simulink model "Aircraft6DOFTrim"  (R2022a)
settings: Solver=VariableStepAuto  StartTime=0.0  StopTime=300  FixedStep=0.5  RelTol=1e-3
undefined symbols (not defined in the file): a0, a1, a2, a3, ac, alpha0, alpha_stall, c, cbar, cg, CLa, delta_aileronMax, delta_aileronMin, delta_elevatorMax, delta_elevatorMin, delta_rudderMax, delta_rudderMin, delta_thrustMax, delta_thrustMin, depsilon, Earth, engArm1, engArm2, falling_slew_rate, h_ref, Lat0, Lon0, LT, mass, rising_slew_rate, S, ST, WGS84, x
libraries: aerolibasang x3, aerolibfltsims x2, aerolibatmos2 x1, aerolibtransform2 x1
settings Model: Creator=wangL  LastModifiedBy=wangL
settings DataIOCC: ExternalInput=U_trim.getElement(1),U_trim.getElement(2),U_trim.getElement(3),U_trim.getElement(4),U_trim.getElement(5)

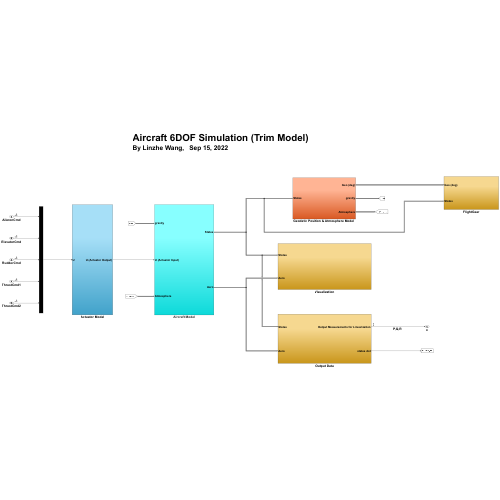
[thumbnail: Simulink's stored preview of the top-level diagram]
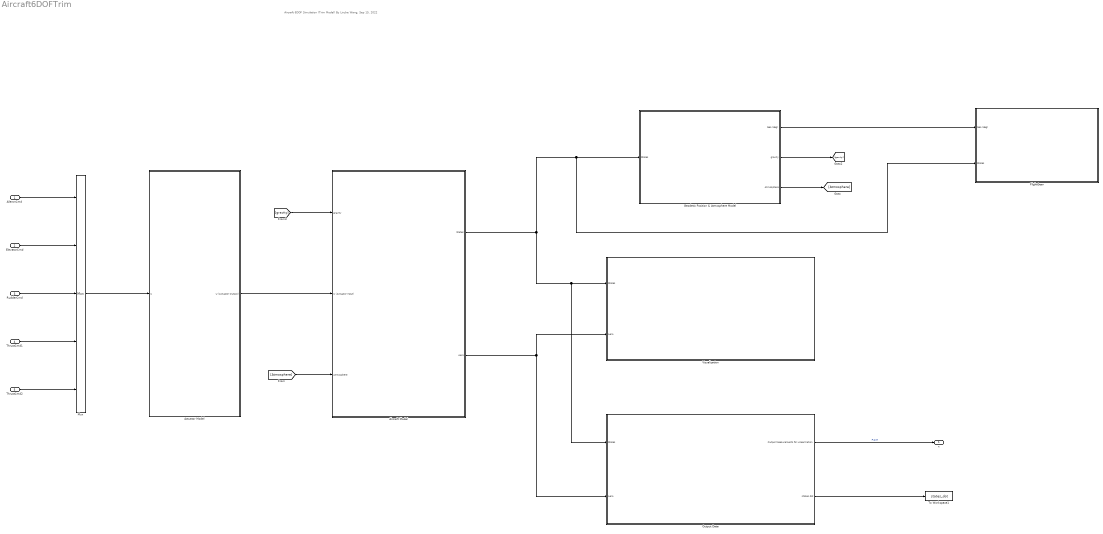
== system Aircraft6DOFTrim ==
  note: Aircraft 6DOF Simulation (Trim Model)
      | By Linzhe Wang, Sep 15, 2022
  AileronCmd : Inport
  ElevatorCmd : Inport  Port=2
  RudderCmd : Inport  Port=3
  ThrustCmd1 : Inport  Port=4
  ThrustCmd2 : Inport  Port=5
  Actuator Model : Subsystem
  Aircraft Model : Subsystem
  FlightGear : Subsystem
  "Geodetic Position & Atmosphere Model " : Subsystem
  Mux : Mux  Inputs=5
  Output Data : Subsystem
  To Workspace1 : ToWorkspace  VariableName=states_dot  SaveFormat=Structure With Time  SampleTime=-1
      settings: MaxDataPoints=1
  Visualization : Subsystem
  x : Outport
  wires:
  "Geodetic Position & Atmosphere Model "/1(Geo (deg)) -> FlightGear/1(Geo (deg))
  "Geodetic Position & Atmosphere Model "/2(gravity) -> [gravity]
  [gravity] -> Aircraft Model/1(gravity)
  Actuator Model/1(U (Actuator Output)) -> Aircraft Model/2(U (Actuator Input))
  "Geodetic Position & Atmosphere Model "/3(Atmosphere) -> [Atmosphere]
  [Atmosphere] -> Aircraft Model/3(Atmosphere)
  ElevatorCmd/1 -> Mux/2
  ThrustCmd2/1 -> Mux/5
  ThrustCmd1/1 -> Mux/4
  Mux/1 -> Actuator Model/1(U)
  RudderCmd/1 -> Mux/3
  AileronCmd/1 -> Mux/1
  Output Data/1(Output Measurements for Linearization) -> x/1  "P,Q,R"
  Output Data/2(states dot) -> To Workspace1/1
  Aircraft Model/1(States) -> Output Data/1(States), Visualization/1(States), "Geodetic Position & Atmosphere Model "/1(States), FlightGear/2(States)
  Aircraft Model/2(Aero) -> Output Data/2(Aero), Visualization/2(Aero)

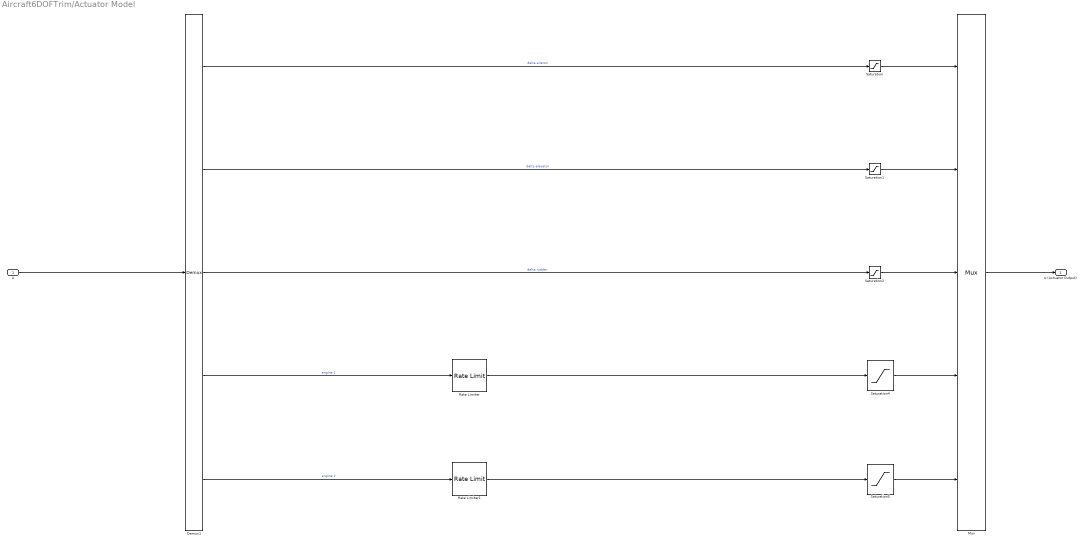
== system Aircraft6DOFTrim/Actuator Model ==
  U : Inport
  Demux1 : Demux  Outputs=5
  Mux : Mux  Inputs=5
  Rate Limiter : RateLimiter  RisingSlewLimit=rising_slew_rate  FallingSlewLimit=falling_slew_rate  SampleTimeMode=inherited
  Rate Limiter1 : RateLimiter  RisingSlewLimit=rising_slew_rate  FallingSlewLimit=falling_slew_rate  SampleTimeMode=inherited
  Saturation : Saturate  UpperLimit=delta_aileronMax  LowerLimit=delta_aileronMin
  Saturation1 : Saturate  UpperLimit=delta_elevatorMax  LowerLimit=delta_elevatorMin
  Saturation2 : Saturate  UpperLimit=delta_rudderMax  LowerLimit=delta_rudderMin
  Saturation4 : Saturate  UpperLimit=delta_thrustMax  LowerLimit=delta_thrustMin
  Saturation5 : Saturate  UpperLimit=delta_thrustMax  LowerLimit=delta_thrustMin
  U (Actuator Output) : Outport
  wires:
  Demux1/3 -> Saturation2/1  "delta rudder"
  Demux1/5 -> Rate Limiter1/1  "engine 2"
  Saturation4/1 -> Mux/4
  Saturation5/1 -> Mux/5
  Mux/1 -> U (Actuator Output)/1
  Demux1/2 -> Saturation1/1  "delta elevator"
  Demux1/1 -> Saturation/1  "delta aileron"
  Saturation/1 -> Mux/1
  Saturation1/1 -> Mux/2
  Saturation2/1 -> Mux/3
  Demux1/4 -> Rate Limiter/1  "engine 1"
  Rate Limiter1/1 -> Saturation5/1
  Rate Limiter/1 -> Saturation4/1
  U/1 -> Demux1/1

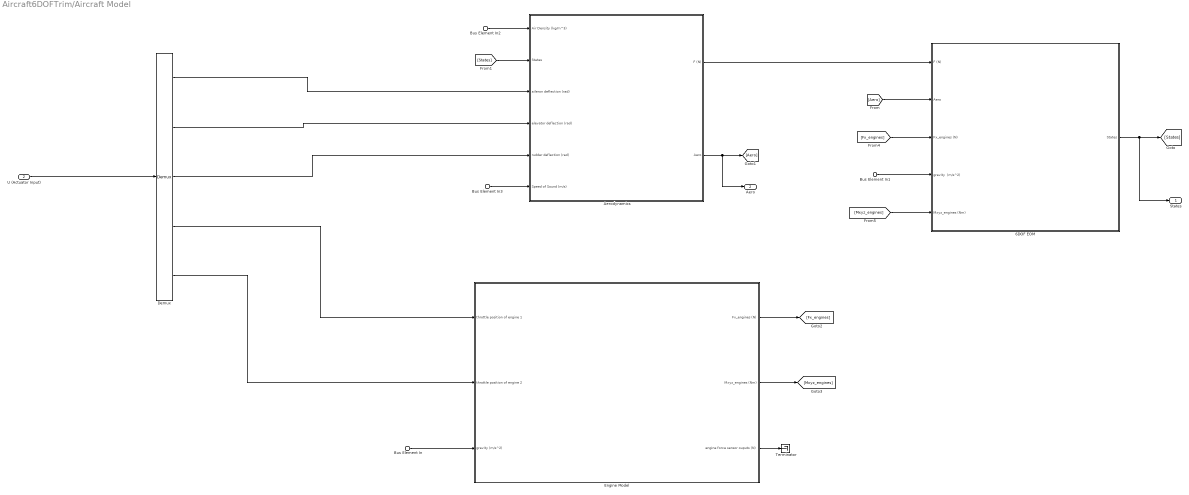
== system Aircraft6DOFTrim/Aircraft Model ==
  Bus Element In : Inport  PortName=gravity  Element=m/s^2
  Bus Element In1 : Inport  PortName=gravity  Element=m/s^2
  U (Actuator Input) : Inport  Port=2
  Bus Element In2 : Inport  Port=3  PortName=Atmosphere  Element=rho
  Bus Element In3 : Inport  Port=3  PortName=Atmosphere  Element=speedOfSound
  6DOF EOM : Subsystem
  Aerodynamics : Subsystem
  Demux : Demux  Outputs=5
  "Engine Model " : Subsystem
  Terminator : Terminator
  States : Outport
  Aero : Outport  Port=2
  wires:
  [Fx_engines] -> 6DOF EOM/3(Fx_engines (N))
  [Mxyz_engines] -> 6DOF EOM/5("Mxyz_engines (Nm) ")
  Aerodynamics/1(F (N)) -> 6DOF EOM/1(F (N))
  6DOF EOM/1(States) -> States/1, [States]
  "Engine Model "/1(Fx_engines (N)) -> [Fx_engines]
  "Engine Model "/2("Mxyz_engines (Nm) ") -> [Mxyz_engines]
  Aerodynamics/2(Aero) -> Aero/1, [Aero]
  [States] -> Aerodynamics/2(States)
  [Aero] -> 6DOF EOM/2(Aero)
  U (Actuator Input)/1 -> Demux/1
  Bus Element In/1 -> "Engine Model "/3(gravity (m/s^2))
  Bus Element In1/1 -> 6DOF EOM/4(gravity  (m/s^2))
  "Engine Model "/3(engine force sensor ouputs (N)) -> Terminator/1
  Demux/1 -> Aerodynamics/3(aileron deflection (rad))
  Demux/2 -> Aerodynamics/4(" elevator deflection (rad)")
  Demux/3 -> Aerodynamics/5(rudder deflection (rad))
  Demux/4 -> "Engine Model "/1(throttle position of engine 1)
  Demux/5 -> "Engine Model "/2(throttle position of engine 2)
  Bus Element In2/1 -> Aerodynamics/1(Air Density (kg/m^3))
  Bus Element In3/1 -> Aerodynamics/6(Speed of Sound (m/s))

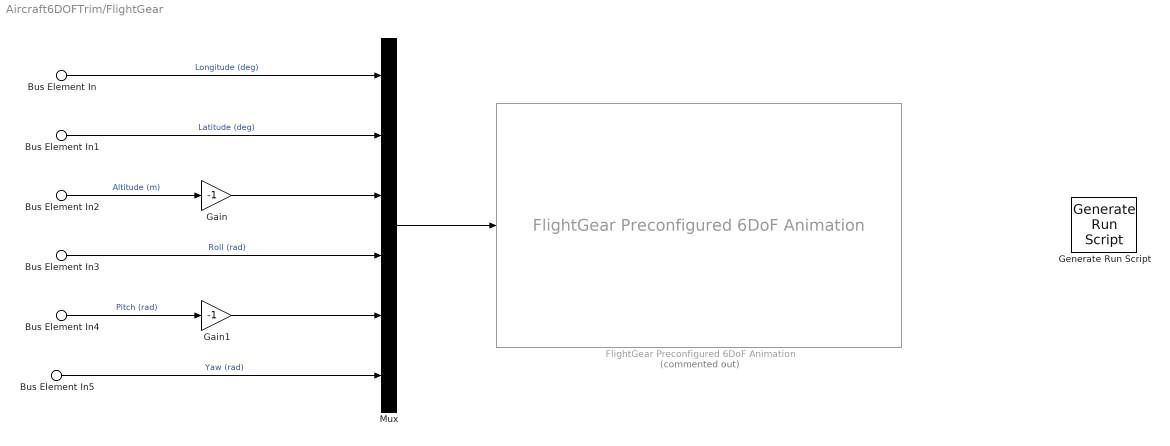
== system Aircraft6DOFTrim/FlightGear ==
  Bus Element In : Inport  PortName=Geo (deg)  Element=Lon
  Bus Element In1 : Inport  PortName=Geo (deg)  Element=Lat
  Bus Element In2 : Inport  Port=2  PortName=States  Element=h
  Bus Element In3 : Inport  Port=2  PortName=States  Element=phi
  Bus Element In4 : Inport  Port=2  PortName=States  Element=theta
  Bus Element In5 : Inport  Port=2  PortName=States  Element=psi
  FlightGear Preconfigured 6DoF Animation : aerolibfltsims/FlightGear Preconfigured 6DoF Animation  Commented=on  xFlightGearVersion=v2019.1  DestinationIpAddress=127.0.0.1  DestinationPort=5502  SampleTime=1/30  packetVersion=24
  Gain : Gain  Gain=-1
  Gain1 : Gain  Gain=-1
  Generate Run Script : aerolibfltsims/Generate Run Script  Architecture=Win64  dataFlow=Send  GeometryModelName=738  AirportId=KSFO  RunwayId=10L  InitialAltitude=0  InitialHeading=0  OffsetDistance=0  OffsetAzimuth=0  InstallScenery=off  DisableShaders=on  OriginAddress=127.0.0.1  DestinationPort=5502  OriginPort=5505  LocalAddress=127.0.0.1  OutputFileName=runfg.bat  FlightGearBaseDirectory=C:\Program Files\FlightGear 2020.3
  Mux : Mux  Inputs=6
  wires:
  Mux/1 -> FlightGear Preconfigured 6DoF Animation/1
  Bus Element In/1 -> Mux/1  "Longitude (deg)"
  Bus Element In1/1 -> Mux/2  "Latitude (deg)"
  Bus Element In2/1 -> Gain/1  "Altitude (m)"
  Bus Element In3/1 -> Mux/4  "Roll (rad)"
  Bus Element In4/1 -> Gain1/1  "Pitch (rad)"
  Bus Element In5/1 -> Mux/6  "Yaw (rad)"
  Gain/1 -> Mux/3
  Gain1/1 -> Mux/5

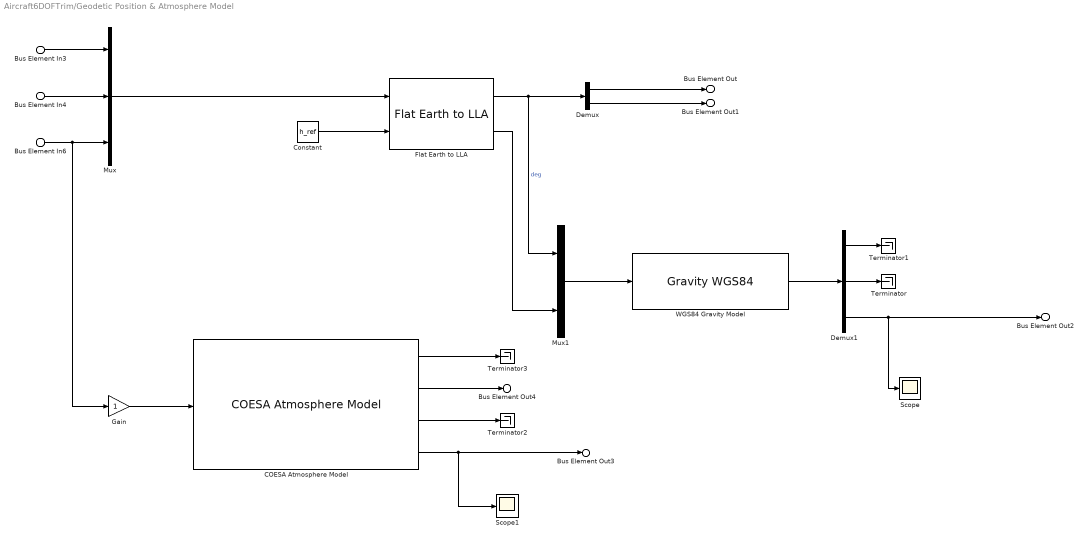
== system Aircraft6DOFTrim/Geodetic Position & Atmosphere Model  ==
  Bus Element In3 : Inport  PortName=States  Element=PN
  Bus Element In4 : Inport  PortName=States  Element=PE
  Bus Element In6 : Inport  PortName=States  Element=h
  COESA Atmosphere Model : aerolibatmos2/COESA Atmosphere Model  units=Metric (MKS)  spec=1976 COESA-extended U.S. Standard Atmosphere  model=Profile  profile_var=High temperature  profile_percent=1%  profile_alt=5 km (16404 ft)  envelope_var=High temperature  envelope_percent=1%  action=None
  Constant : Constant  Value=h_ref
  Demux : Demux  Outputs=2
  Demux1 : Demux  Outputs=3
  Flat Earth to LLA : aerolibtransform2/Flat Earth to LLA  units=Metric (MKS)  ptype=Earth (WGS84)  F=1/298.257223563  R=6378137  refPosPort=off  LL0=[Lat0 Lon0]  psi=0
  Gain : Gain
  Mux : Mux  Inputs=3
  Mux1 : Mux  Inputs=2
  Scope : Scope
  Scope1 : Scope
  Terminator{,1..3} (4 alike) : Terminator
  "WGS84 Gravity Model  " : GravityWGS84  action=None
  Bus Element Out : Outport  PortName=Geo (deg)  Element=Lat
  Bus Element Out1 : Outport  PortName=Geo (deg)  Element=Lon
  Bus Element Out2 : Outport  Port=2  PortName=gravity  Element=m/s^2
  Bus Element Out3 : Outport  Port=3  PortName=Atmosphere  Element=rho
  Bus Element Out4 : Outport  Port=3  PortName=Atmosphere  Element=speedOfSound
  wires:
  Constant/1 -> Flat Earth to LLA/2
  Bus Element In3/1 -> Mux/1
  Bus Element In4/1 -> Mux/2
  Bus Element In6/1 -> Mux/3, Gain/1
  Flat Earth to LLA/1 -> Demux/1, Mux1/1  "deg"
  Demux/1 -> Bus Element Out/1
  Demux/2 -> Bus Element Out1/1
  Mux/1 -> Flat Earth to LLA/1
  Mux1/1 -> "WGS84 Gravity Model  "/1
  Flat Earth to LLA/2 -> Mux1/2
  "WGS84 Gravity Model  "/1 -> Demux1/1
  Demux1/2 -> Terminator/1
  Demux1/1 -> Terminator1/1
  Demux1/3 -> Bus Element Out2/1, Scope/1
  COESA Atmosphere Model/2 -> Bus Element Out4/1
  COESA Atmosphere Model/3 -> Terminator2/1
  COESA Atmosphere Model/1 -> Terminator3/1
  Gain/1 -> COESA Atmosphere Model/1
  COESA Atmosphere Model/4 -> Bus Element Out3/1, Scope1/1

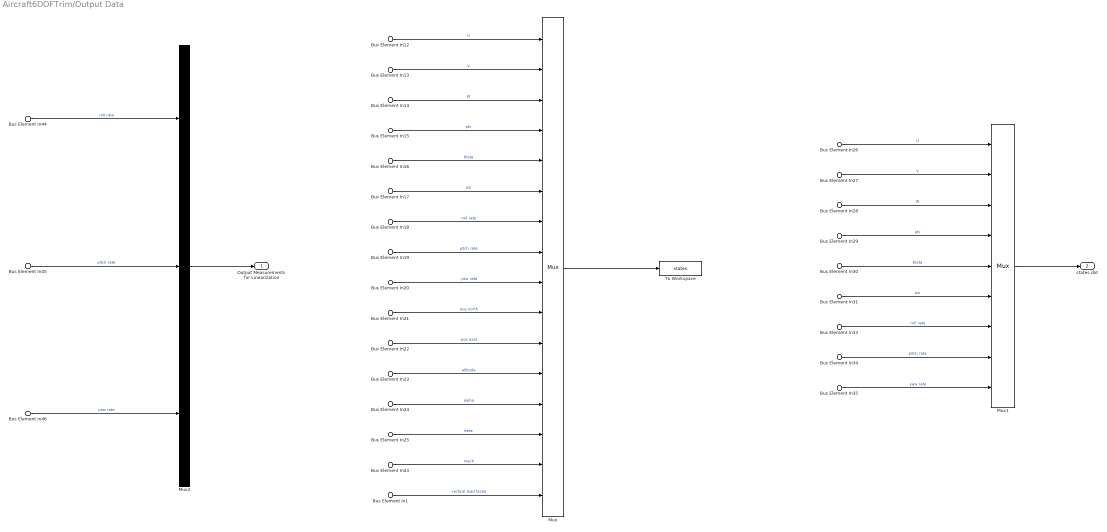
== system Aircraft6DOFTrim/Output Data ==
  Bus Element In12 : Inport  PortName=States  Element=U
  Bus Element In13 : Inport  PortName=States  Element=V
  Bus Element In14 : Inport  PortName=States  Element=W
  Bus Element In15 : Inport  PortName=States  Element=phi
  Bus Element In16 : Inport  PortName=States  Element=theta
  Bus Element In17 : Inport  PortName=States  Element=psi
  Bus Element In44 : Inport  PortName=States  Element=P
  Bus Element In18 : Inport  PortName=States  Element=P
  Bus Element In45 : Inport  PortName=States  Element=Q
  Bus Element In19 : Inport  PortName=States  Element=Q
  Bus Element In46 : Inport  PortName=States  Element=R
  Bus Element In20 : Inport  PortName=States  Element=R
  Bus Element In26 : Inport  PortName=States  Element=U_dot
  Bus Element In27 : Inport  PortName=States  Element=V_dot
  Bus Element In28 : Inport  PortName=States  Element=W_dot
  Bus Element In29 : Inport  PortName=States  Element=phi_dot
  Bus Element In30 : Inport  PortName=States  Element=theta_dot
  Bus Element In31 : Inport  PortName=States  Element=psi_dot
  Bus Element In33 : Inport  PortName=States  Element=P_dot
  Bus Element In34 : Inport  PortName=States  Element=Q_dot
  Bus Element In35 : Inport  PortName=States  Element=R_dot
  Bus Element In23 : Inport  PortName=States  Element=h
  Bus Element In21 : Inport  PortName=States  Element=PN
  Bus Element In22 : Inport  PortName=States  Element=PE
  Bus Element In1 : Inport  PortName=States  Element=Nz
  Bus Element In24 : Inport  Port=2  PortName=Aero  Element=alpha
  Bus Element In25 : Inport  Port=2  PortName=Aero  Element=beta
  Bus Element In43 : Inport  Port=2  PortName=Aero  Element=mach
  Mux : Mux  Inputs=16
  Mux1 : Mux  Inputs=9
  Mux2 : Mux  Inputs=3
  To Workspace : ToWorkspace  VariableName=states  SaveFormat=Structure With Time  SampleTime=-1
  Output Measurements for Linearization : Outport
  states dot : Outport  Port=2
  wires:
  Mux/1 -> To Workspace/1
  Bus Element In26/1 -> Mux1/1  "U"
  Bus Element In30/1 -> Mux1/5  "theta"
  Bus Element In29/1 -> Mux1/4  "phi"
  Bus Element In27/1 -> Mux1/2  "V"
  Bus Element In28/1 -> Mux1/3  "W"
  Bus Element In31/1 -> Mux1/6  "psi"
  Bus Element In33/1 -> Mux1/7  "roll rate"
  Bus Element In34/1 -> Mux1/8  "pitch rate"
  Bus Element In35/1 -> Mux1/9  "yaw rate"
  Mux1/1 -> states dot/1
  Bus Element In45/1 -> Mux2/2  "pitch rate"
  Mux2/1 -> Output Measurements for Linearization/1
  Bus Element In46/1 -> Mux2/3  "yaw rate"
  Bus Element In44/1 -> Mux2/1  "roll rate"
  Bus Element In1/1 -> Mux/16  "vertical load factor"
  Bus Element In43/1 -> Mux/15  "mach"
  Bus Element In23/1 -> Mux/12  "altitude"
  Bus Element In14/1 -> Mux/3  "W"
  Bus Element In13/1 -> Mux/2  "V"
  Bus Element In12/1 -> Mux/1  "U"
  Bus Element In17/1 -> Mux/6  "psi"
  Bus Element In18/1 -> Mux/7  "roll rate"
  Bus Element In19/1 -> Mux/8  "pitch rate"
  Bus Element In16/1 -> Mux/5  "theta"
  Bus Element In15/1 -> Mux/4  "phi"
  Bus Element In22/1 -> Mux/11  "pos east"
  Bus Element In25/1 -> Mux/14  "beta"
  Bus Element In24/1 -> Mux/13  "alpha"
  Bus Element In20/1 -> Mux/9  "yaw rate"
  Bus Element In21/1 -> Mux/10  "pos north"

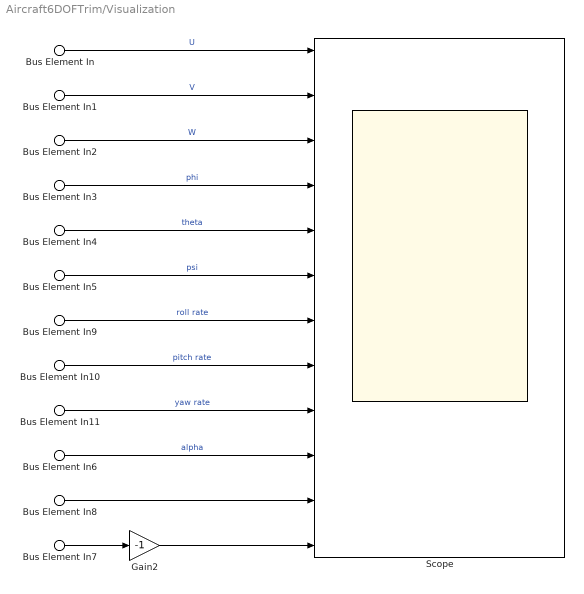
== system Aircraft6DOFTrim/Visualization ==
  Bus Element In : Inport  PortName=States  Element=U
  Bus Element In1 : Inport  PortName=States  Element=V
  Bus Element In2 : Inport  PortName=States  Element=W
  Bus Element In3 : Inport  PortName=States  Element=phi
  Bus Element In4 : Inport  PortName=States  Element=theta
  Bus Element In5 : Inport  PortName=States  Element=psi
  Bus Element In7 : Inport  PortName=States  Element=h
  Bus Element In9 : Inport  PortName=States  Element=P
  Bus Element In10 : Inport  PortName=States  Element=Q
  Bus Element In11 : Inport  PortName=States  Element=R
  Bus Element In6 : Inport  Port=2  PortName=Aero  Element=alpha
  Bus Element In8 : Inport  Port=2  PortName=Aero  Element=beta
  Gain2 : Gain  Gain=-1
  Scope : Scope  NumInputPorts=12
  wires:
  Bus Element In5/1 -> Scope/6  "psi"
  Bus Element In11/1 -> Scope/9  "yaw rate"
  Bus Element In2/1 -> Scope/3  "W"
  Bus Element In1/1 -> Scope/2  "V"
  Bus Element In10/1 -> Scope/8  "pitch rate"
  Bus Element In/1 -> Scope/1  "U"
  Gain2/1 -> Scope/12
  Bus Element In9/1 -> Scope/7  "roll rate"
  Bus Element In6/1 -> Scope/10  "alpha"
  Bus Element In4/1 -> Scope/5  "theta"
  Bus Element In8/1 -> Scope/11
  Bus Element In3/1 -> Scope/4  "phi"
  Bus Element In7/1 -> Gain2/1

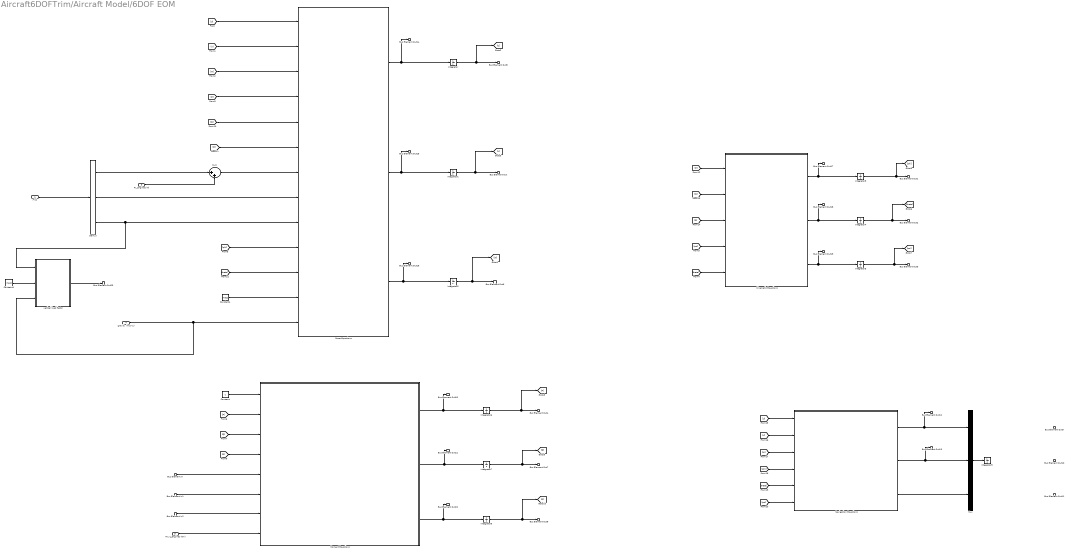
== system Aircraft6DOFTrim/Aircraft Model/6DOF EOM ==
  F (N) : Inport
  Bus Element In : Inport  Port=2  PortName=Aero  Element=L_roll
  Bus Element In1 : Inport  Port=2  PortName=Aero  Element=M_pitch
  Bus Element In2 : Inport  Port=2  PortName=Aero  Element=N_yaw
  Fx_engines (N) : Inport  Port=3
  gravity  (m/s^2) : Inport  Port=4
  "Mxyz_engines (Nm) " : Inport  Port=5
  Constant : Constant  Value=c
  Constant1 : Constant  Value=mass
  Constant4 : Constant  Value=mass
  Demux : Demux  Outputs=3
  Force Equations : MATLAB Function  TreatAsAtomicUnit=on
  Integrator : Integrator  InitialCondition=x(1)  ContinuousStateAttributes='U'
  Integrator1 : Integrator  InitialCondition=x(2)  ContinuousStateAttributes='V'
  Integrator2 : Integrator  InitialCondition=x(3)  ContinuousStateAttributes='W'
  Integrator3 : Integrator  InitialCondition=x(4)  WrapState=on  ContinuousStateAttributes='phi'
  Integrator4 : Integrator  InitialCondition=x(5)  WrapState=on  ContinuousStateAttributes='theta'
  Integrator5 : Integrator  InitialCondition=x(6)  WrapState=on  ContinuousStateAttributes='psi'
  Integrator6 : Integrator  InitialCondition=x(7)  ContinuousStateAttributes='P'
  Integrator7 : Integrator  InitialCondition=x(8)  ContinuousStateAttributes='Q'
  Integrator8 : Integrator  InitialCondition=x(9)  ContinuousStateAttributes='R'
  Integrator9 : Integrator  InitialCondition=x(10:12)  ContinuousStateAttributes='PN_PE_h'
  Kinematic Equations : MATLAB Function  TreatAsAtomicUnit=on
  Moment Equations : MATLAB Function  TreatAsAtomicUnit=on
  Mux : Mux  Inputs=3
  Navigation Equations : MATLAB Function  TreatAsAtomicUnit=on
  Sum : Sum  Inputs=|++
  vertical load factor : MATLAB Function  TreatAsAtomicUnit=on
  Bus Element Out : Outport  VectorParamsAs1DForOutWhenUnconnected=off  PortName=States  Element=V
  Bus Element Out5 : Outport  VectorParamsAs1DForOutWhenUnconnected=off  PortName=States  Element=U
  Bus Element Out6 : Outport  VectorParamsAs1DForOutWhenUnconnected=off  PortName=States  Element=W
  Bus Element Out1 : Outport  VectorParamsAs1DForOutWhenUnconnected=off  PortName=States  Element=phi
  Bus Element Out2 : Outport  VectorParamsAs1DForOutWhenUnconnected=off  PortName=States  Element=theta
  Bus Element Out3 : Outport  VectorParamsAs1DForOutWhenUnconnected=off  PortName=States  Element=psi
  Bus Element Out4 : Outport  VectorParamsAs1DForOutWhenUnconnected=off  PortName=States  Element=P
  Bus Element Out7 : Outport  VectorParamsAs1DForOutWhenUnconnected=off  PortName=States  Element=Q
  Bus Element Out8 : Outport  VectorParamsAs1DForOutWhenUnconnected=off  PortName=States  Element=R
  Bus Element Out9 : Outport  VectorParamsAs1DForOutWhenUnconnected=off  PortName=States  Element=PN
  Bus Element Out10 : Outport  VectorParamsAs1DForOutWhenUnconnected=off  PortName=States  Element=PE
  Bus Element Out11 : Outport  VectorParamsAs1DForOutWhenUnconnected=off  PortName=States  Element=h
  Bus Element Out12 : Outport  VectorParamsAs1DForOutWhenUnconnected=off  PortName=States  Element=PN_dot
  Bus Element Out13 : Outport  VectorParamsAs1DForOutWhenUnconnected=off  PortName=States  Element=PE_dot
  Bus Element Out14 : Outport  VectorParamsAs1DForOutWhenUnconnected=off  PortName=States  Element=U_dot
  Bus Element Out15 : Outport  VectorParamsAs1DForOutWhenUnconnected=off  PortName=States  Element=V_dot
  Bus Element Out16 : Outport  VectorParamsAs1DForOutWhenUnconnected=off  PortName=States  Element=W_dot
  Bus Element Out17 : Outport  VectorParamsAs1DForOutWhenUnconnected=off  PortName=States  Element=phi_dot
  Bus Element Out18 : Outport  VectorParamsAs1DForOutWhenUnconnected=off  PortName=States  Element=theta_dot
  Bus Element Out19 : Outport  VectorParamsAs1DForOutWhenUnconnected=off  PortName=States  Element=psi_dot
  Bus Element Out20 : Outport  VectorParamsAs1DForOutWhenUnconnected=off  PortName=States  Element=P_dot
  Bus Element Out21 : Outport  VectorParamsAs1DForOutWhenUnconnected=off  PortName=States  Element=Q_dot
  Bus Element Out22 : Outport  VectorParamsAs1DForOutWhenUnconnected=off  PortName=States  Element=R_dot
  Bus Element Out23 : Outport  VectorParamsAs1DForOutWhenUnconnected=off  PortName=States  Element=Nz
  wires:
  F (N)/1 -> Demux/1
  Force Equations/1(U_dot) -> Integrator/1, Bus Element Out14/1
  Force Equations/3(W_dot) -> Integrator2/1, Bus Element Out16/1
  Force Equations/2(V_dot) -> Bus Element Out15/1, Integrator1/1
  Integrator1/1 -> [V], Bus Element Out/1
  Integrator/1 -> [U], Bus Element Out5/1
  Integrator2/1 -> Bus Element Out6/1, [W]
  [U] -> Force Equations/1(U)
  [V] -> Force Equations/2(V)
  [W] -> Force Equations/3(W)
  Kinematic Equations/1(phi_dot) -> Bus Element Out17/1, Integrator3/1
  Kinematic Equations/2(theta_dot) -> Integrator4/1, Bus Element Out18/1
  Kinematic Equations/3(psi_dot) -> Bus Element Out19/1, Integrator5/1
  Integrator3/1 -> [phi], Bus Element Out1/1
  Integrator4/1 -> Bus Element Out2/1, [theta]
  Integrator5/1 -> [psi], Bus Element Out3/1
  [psi] -> Kinematic Equations/4(phi)
  [theta] -> Kinematic Equations/5(theta)
  [phi] -> Force Equations/10(phi)
  Moment Equations/1(P_dot) -> Integrator6/1, Bus Element Out20/1
  Moment Equations/2(Q_dot) -> Integrator7/1, Bus Element Out21/1
  Moment Equations/3(R_dot) -> Integrator8/1, Bus Element Out22/1
  Integrator6/1 -> Bus Element Out4/1, [P]
  Integrator7/1 -> [Q], Bus Element Out7/1
  Integrator8/1 -> [R], Bus Element Out8/1
  [P] -> Moment Equations/2(P)
  [Q] -> Moment Equations/3(Q)
  [R] -> Moment Equations/4(R)
  [P] -> Force Equations/4(P)
  [Q] -> Force Equations/5(Q)
  [R] -> Force Equations/6(R)
  [P] -> Kinematic Equations/1(P)
  [Q] -> Kinematic Equations/2(Q)
  [R] -> Kinematic Equations/3(R)
  Constant4/1 -> Force Equations/12(m)
  [U] -> Navigation Equations/1(U)
  [V] -> Navigation Equations/2(V)
  [W] -> Navigation Equations/3(W)
  [phi] -> Navigation Equations/4(phi)
  [theta] -> Navigation Equations/5(theta)
  [psi] -> Navigation Equations/6(psi)
  Navigation Equations/1(PN_dot) -> Mux/1, Bus Element Out12/1
  Navigation Equations/2(PE_dot) -> Mux/2, Bus Element Out13/1
  Bus Element In/1 -> Moment Equations/5(L_roll)
  Bus Element In1/1 -> Moment Equations/6(M_pitch)
  Bus Element In2/1 -> Moment Equations/7(N_yaw)
  Demux/2 -> Force Equations/8(Fy)
  [theta] -> Force Equations/11(theta)
  Constant/1 -> Moment Equations/1(c)
  Demux/1 -> Sum/1
  Sum/1 -> Force Equations/7(Fx)
  Fx_engines (N)/1 -> Sum/2
  "Mxyz_engines (Nm) "/1 -> Moment Equations/8(Mxyz_engines)
  gravity  (m/s^2)/1 -> vertical load factor/3(g), Force Equations/13(g)
  Demux/3 -> vertical load factor/1(Fz), Force Equations/9(Fz)
  Constant1/1 -> vertical load factor/2(mass)
  vertical load factor/1(Nz) -> Bus Element Out23/1
  Navigation Equations/3(h_dot) -> Mux/3
  ? -> Bus Element Out11/1
  ? -> Bus Element Out9/1
  ? -> Bus Element Out10/1
  Mux/1 -> Integrator9/1

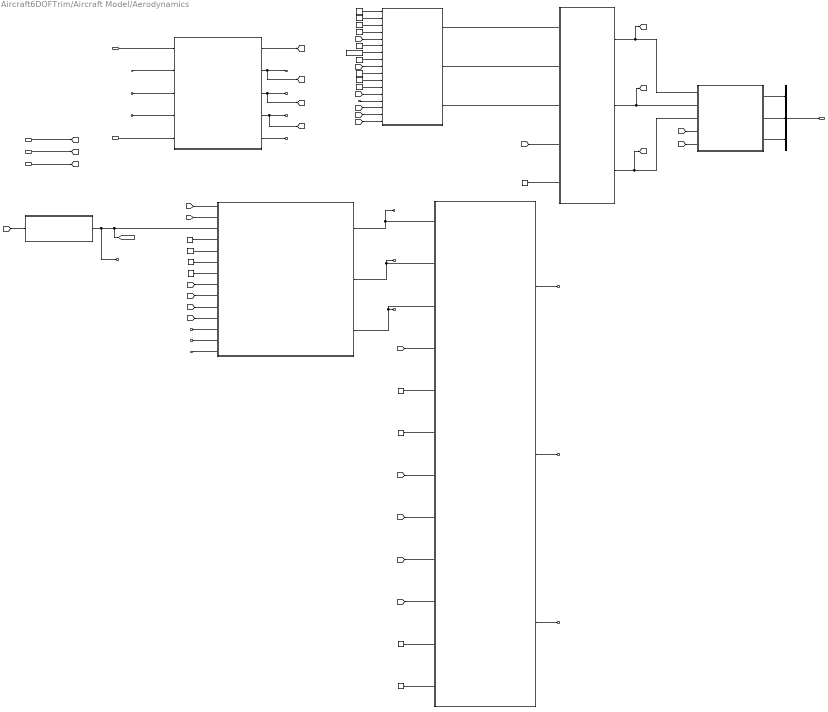
== system Aircraft6DOFTrim/Aircraft Model/Aerodynamics ==
  Air Density (kg/m^3) : Inport
  Bus Element In2 : Inport  Port=2  PortName=States  Element=P
  Bus Element In3 : Inport  Port=2  PortName=States  Element=Q
  Bus Element In7 : Inport  Port=2  PortName=States  Element=Q
  Bus Element In4 : Inport  Port=2  PortName=States  Element=R
  Bus Element In1 : Inport  Port=2  PortName=States  Element=U
  Bus Element In5 : Inport  Port=2  PortName=States  Element=W
  Bus Element In6 : Inport  Port=2  PortName=States  Element=V
  aileron deflection (rad) : Inport  Port=3
  " elevator deflection (rad)" : Inport  Port=4
  rudder deflection (rad) : Inport  Port=5
  Speed of Sound (m/s) : Inport  Port=6
  Aerodynamic Coefficients : MATLAB Function  TreatAsAtomicUnit=on
  Aerodynamic Force : MATLAB Function  TreatAsAtomicUnit=on
  Aerodynamic Force in Body-axes : MATLAB Function  TreatAsAtomicUnit=on
  Constant : Constant  Value=S
  Constant1 : Constant  Value=cg
  Constant10 : Constant  Value=a0
  Constant11 : Constant  Value=a1
  Constant12 : Constant  Value=a2
  Constant13 : Constant  Value=a3
  Constant14 : Constant  Value=ac
  Constant2 : Constant  Value=cbar
  Constant3 : Constant  Value=alpha0
  Constant4 : Constant  Value=ST
  Constant5 : Constant  Value=S
  Constant6 : Constant  Value=LT
  Constant7 : Constant  Value=S
  Constant8 : Constant  Value=CLa
  Constant9 : Constant  Value=alpha_stall
  Moment Calculations : MATLAB Function  TreatAsAtomicUnit=on
  Moment Coefficients : MATLAB Function  TreatAsAtomicUnit=on
  Mux : Mux  Inputs=3
  Subsystem : Subsystem
  dist CG and Tail_ac (m) : Constant  Value=LT
  downwash angle : Subsystem
  generalised length (m) : Constant  Value=cbar
  tail planform area (m^2) : Constant  Value=ST
  wing planform area (m^2) : Constant  Value=S
  F (N) : Outport
  Bus Element Out : Outport  Port=2  PortName=Aero  Element=L_roll
  Bus Element Out1 : Outport  Port=2  PortName=Aero  Element=M_pitch
  Bus Element Out2 : Outport  Port=2  PortName=Aero  Element=N_yaw
  Bus Element Out3 : Outport  Port=2  PortName=Aero  Element=alpha
  Bus Element Out4 : Outport  Port=2  PortName=Aero  Element=beta
  Bus Element Out5 : Outport  Port=2  PortName=Aero  Element=V_tot
  Bus Element Out6 : Outport  Port=2  PortName=Aero  Element=epsilon
  Bus Element Out7 : Outport  Port=2  PortName=Aero  Element=Cl
  Bus Element Out8 : Outport  Port=2  PortName=Aero  Element=Cm
  Bus Element Out9 : Outport  Port=2  PortName=Aero  Element=Cn
  Bus Element Out10 : Outport  Port=2  PortName=Aero  Element=mach
  wires:
  Air Density (kg/m^3)/1 -> Subsystem/1(Air Density (kg/m^3))
  Moment Coefficients/1(Cl) -> Bus Element Out7/1, Moment Calculations/1(Cl)
  Moment Coefficients/2(Cm) -> Bus Element Out8/1, Moment Calculations/2(Cm)
  Moment Coefficients/3(Cn) -> Bus Element Out9/1, Moment Calculations/3(Cn)
  Moment Calculations/1(L_roll) -> Bus Element Out/1
  Moment Calculations/2(M_pitch) -> Bus Element Out1/1
  Moment Calculations/3(N_yaw) -> Bus Element Out2/1
  tail planform area (m^2)/1 -> Moment Coefficients/4(ST)
  generalised length (m)/1 -> Moment Coefficients/5(cbar)
  dist CG and Tail_ac (m)/1 -> Moment Coefficients/6(LT)
  Bus Element In2/1 -> Moment Coefficients/12(P)
  Bus Element In3/1 -> Moment Coefficients/13(Q)
  Bus Element In4/1 -> Moment Coefficients/14(R)
  Bus Element In1/1 -> Subsystem/2(U (m/s))
  Bus Element In5/1 -> Subsystem/3(W (m/s))
  Subsystem/1(q_bar (N/m^2)) -> [q_bar]
  Subsystem/2(alpha (rad)) -> [alpha], Bus Element Out3/1
  Subsystem/3(V_tot (m/s)) -> [V_tot], Bus Element Out5/1
  Subsystem/4(beta (rad)) -> [beta], Bus Element Out4/1
  [alpha] -> Moment Coefficients/1(alpha)
  [beta] -> Moment Coefficients/2(beta)
  [V_tot] -> Moment Coefficients/8(V_tot)
  [q_bar] -> Moment Calculations/4(q_bar)
  Constant/1 -> Moment Calculations/5(S)
  Constant2/1 -> Moment Calculations/6(cbar)
  aileron deflection (rad)/1 -> [da]
  " elevator deflection (rad)"/1 -> [de]
  rudder deflection (rad)/1 -> [dr]
  [da] -> Moment Coefficients/9(da)
  [de] -> Moment Coefficients/10(de)
  [dr] -> Moment Coefficients/11(dr)
  downwash angle/1(epsilon (rad)) -> Bus Element Out6/1, Moment Coefficients/3(epsilon), [epsilon]
  [alpha] -> downwash angle/1(alpha (rad))
  [alpha] -> Aerodynamic Coefficients/5(alpha)
  Constant3/1 -> Aerodynamic Coefficients/6(alpha0)
  [beta] -> Aerodynamic Coefficients/9(beta)
  Constant4/1 -> Aerodynamic Coefficients/10(ST)
  Constant5/1 -> Aerodynamic Coefficients/11(S)
  Constant6/1 -> Aerodynamic Coefficients/12(LT)
  [epsilon] -> Aerodynamic Coefficients/13(epsilon)
  Bus Element In6/1 -> Subsystem/4(V (m/s))
  Bus Element In7/1 -> Aerodynamic Coefficients/14(Q)
  [V_tot] -> Aerodynamic Coefficients/15(V_tot)
  [de] -> Aerodynamic Coefficients/16(de)
  [dr] -> Aerodynamic Coefficients/17(dr)
  Aerodynamic Coefficients/1(CL) -> Aerodynamic Force/1(CL)
  Aerodynamic Coefficients/2(CD) -> Aerodynamic Force/2(CD)
  Aerodynamic Coefficients/3(CY) -> Aerodynamic Force/3(CY)
  [q_bar] -> Aerodynamic Force/4(q_bar)
  Constant7/1 -> Aerodynamic Force/5(S)
  Aerodynamic Force/2(D) -> [D], Aerodynamic Force in Body-axes/2(D)
  Aerodynamic Force/1(L) -> [L], Aerodynamic Force in Body-axes/1(L)
  Aerodynamic Force/3(Y) -> [Y], Aerodynamic Force in Body-axes/3(Y)
  [alpha] -> Aerodynamic Force in Body-axes/4(alpha)
  [beta] -> Aerodynamic Force in Body-axes/5(beta)
  Aerodynamic Force in Body-axes/1(Fx) -> Mux/1
  Aerodynamic Force in Body-axes/2(Fy) -> Mux/2
  Aerodynamic Force in Body-axes/3(Fz) -> Mux/3
  Mux/1 -> F (N)/1
  wing planform area (m^2)/1 -> Moment Coefficients/7(S)
  Constant8/1 -> Aerodynamic Coefficients/8(CLa)
  Constant9/1 -> Aerodynamic Coefficients/7(alpha_stall)
  Constant10/1 -> Aerodynamic Coefficients/1(a0)
  Constant11/1 -> Aerodynamic Coefficients/2(a1)
  Constant12/1 -> Aerodynamic Coefficients/3(a2)
  Constant13/1 -> Aerodynamic Coefficients/4(a3)
  [L] -> Moment Calculations/7(L)
  [D] -> Moment Calculations/8(D)
  [Y] -> Moment Calculations/9(Y)
  [alpha] -> Moment Calculations/10(alpha)
  Constant1/1 -> Moment Calculations/11(cg)
  Constant14/1 -> Moment Calculations/12(ac)
  Subsystem/5(Mach) -> Bus Element Out10/1
  Speed of Sound (m/s)/1 -> Subsystem/5("Speed of Sound (m/s) ")

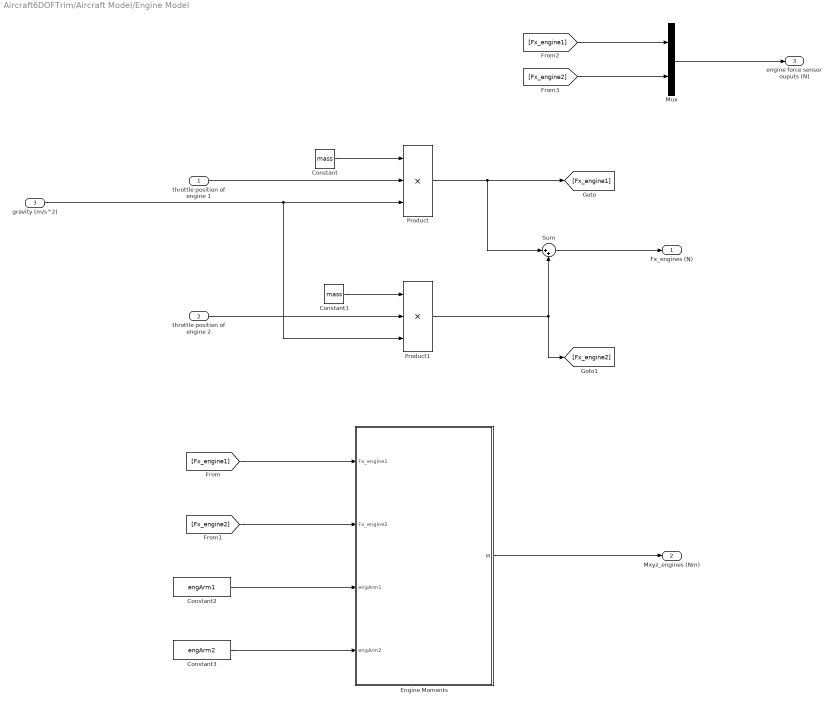
== system Aircraft6DOFTrim/Aircraft Model/Engine Model  ==
  throttle position of engine 1 : Inport
  throttle position of engine 2 : Inport  Port=2
  gravity (m/s^2) : Inport  Port=3
  Constant : Constant  Value=mass
  Constant1 : Constant  Value=mass
  Constant2 : Constant  Value=engArm1
  Constant3 : Constant  Value=engArm2
  Engine Moments : MATLAB Function  TreatAsAtomicUnit=on
  Mux : Mux  Inputs=2
  Product : Product  Inputs=3
  Product1 : Product  Inputs=3
  Sum : Sum  Inputs=|++
  Fx_engines (N) : Outport
  "Mxyz_engines (Nm) " : Outport  Port=2
  engine force sensor ouputs (N) : Outport  Port=3
  wires:
  throttle position of engine 2/1 -> Product1/2
  throttle position of engine 1/1 -> Product/2
  Constant/1 -> Product/1
  Constant1/1 -> Product1/1
  Product/1 -> [Fx_engine1], Sum/1
  Product1/1 -> [Fx_engine2], Sum/2
  Sum/1 -> Fx_engines (N)/1
  gravity (m/s^2)/1 -> Product/3, Product1/3
  [Fx_engine1] -> Engine Moments/1(Fx_engine1)
  [Fx_engine2] -> Engine Moments/2(Fx_engine2)
  Constant2/1 -> Engine Moments/3(engArm1)
  Constant3/1 -> Engine Moments/4(engArm2)
  Engine Moments/1(M) -> "Mxyz_engines (Nm) "/1
  Mux/1 -> engine force sensor ouputs (N)/1
  [Fx_engine1] -> Mux/1
  [Fx_engine2] -> Mux/2

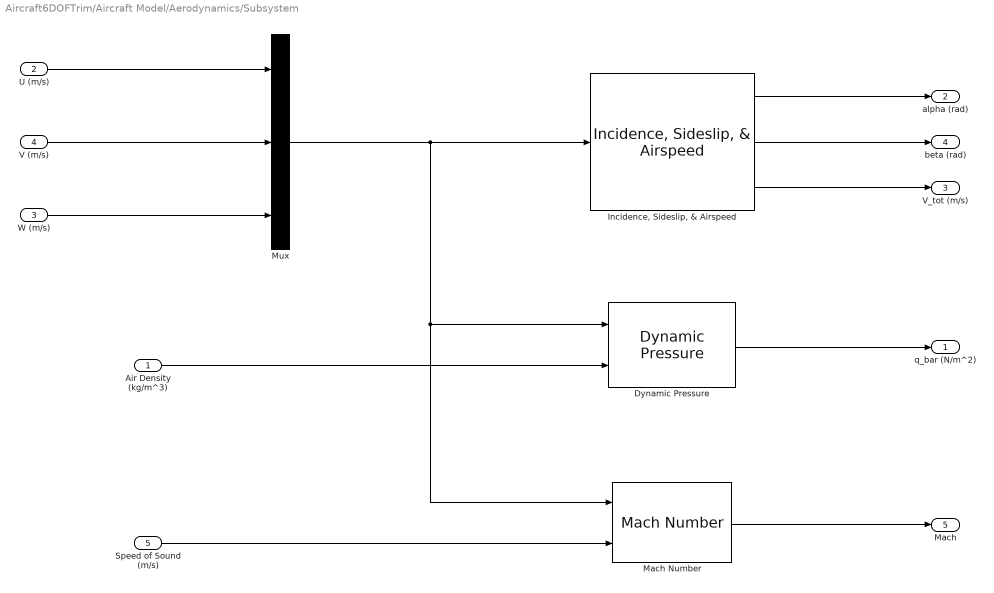
== system Aircraft6DOFTrim/Aircraft Model/Aerodynamics/Subsystem ==
  Air Density (kg/m^3) : Inport
  U (m/s) : Inport  Port=2
  W (m/s) : Inport  Port=3
  V (m/s) : Inport  Port=4
  "Speed of Sound (m/s) " : Inport  Port=5
  Dynamic Pressure : aerolibasang/Dynamic Pressure
  "Incidence, Sideslip, & Airspeed" : aerolibasang/Incidence, Sideslip, & Airspeed
  Mach Number : aerolibasang/Mach Number
      settings: SourceProductBaseCode=AE
  Mux : Mux  Inputs=3
  q_bar (N/m^2) : Outport
  alpha (rad) : Outport  Port=2
  V_tot (m/s) : Outport  Port=3
  beta (rad) : Outport  Port=4
  Mach : Outport  Port=5
  wires:
  "Incidence, Sideslip, & Airspeed"/1 -> alpha (rad)/1
  Dynamic Pressure/1 -> q_bar (N/m^2)/1
  Air Density (kg/m^3)/1 -> Dynamic Pressure/2
  "Incidence, Sideslip, & Airspeed"/2 -> beta (rad)/1
  "Incidence, Sideslip, & Airspeed"/3 -> V_tot (m/s)/1
  U (m/s)/1 -> Mux/1
  V (m/s)/1 -> Mux/2
  W (m/s)/1 -> Mux/3
  Mux/1 -> "Incidence, Sideslip, & Airspeed"/1, Dynamic Pressure/1, Mach Number/1
  "Speed of Sound (m/s) "/1 -> Mach Number/2
  Mach Number/1 -> Mach/1

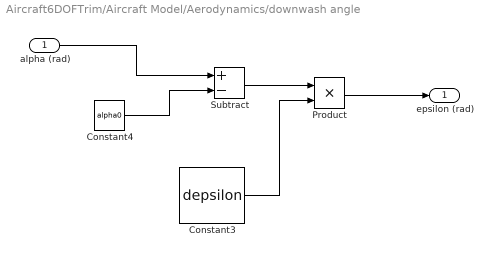
== system Aircraft6DOFTrim/Aircraft Model/Aerodynamics/downwash angle ==
  alpha (rad) : Inport
  Constant3 : Constant  Value=depsilon
  Constant4 : Constant  Value=alpha0
  Product : Product
  Subtract : Sum  Inputs=+-
  epsilon (rad) : Outport
  wires:
  Constant3/1 -> Product/2
  Constant4/1 -> Subtract/2
  alpha (rad)/1 -> Subtract/1
  Subtract/1 -> Product/1
  Product/1 -> epsilon (rad)/1

== matlab function Aircraft6DOFTrim/Aircraft Model/6DOF EOM/Navigation Equations ==
  data: U input; PN_dot output; V input; W input; phi input; theta input; psi input; PE_dot output; h_dot output
function [PN_dot,PE_dot,h_dot] = fcn(U,V,W,phi,theta,psi)

PN_dot = U * cos(theta) * cos(psi) + V * (-cos(phi) * sin(psi) + sin(phi)...
         * sin(theta) * cos(psi)) + W * (sin(phi) * sin(psi) + cos(phi)*...
         sin(theta) * cos(psi));

PE_dot = U * cos(theta) * sin(psi) + V * (cos(phi) * cos(psi) + sin(phi)...
         * sin(theta) * sin(psi)) + W * (-sin(phi) * cos(psi) + cos(phi)...
         * sin(theta) * sin(psi));

h_dot = U * sin(theta) - V * sin(phi) * cos(theta) - W * cos(phi) * cos(theta);

== matlab function Aircraft6DOFTrim/Aircraft Model/Aerodynamics/Moment Coefficients ==
  data: alpha input; Cl output; beta input; epsilon input; ST input; cbar input; LT input; S input; V_tot input; da input; de input; dr input; P input; Q input; R input; Cm output; Cn output
function [Cl,Cm,Cn] = fcn(alpha,beta,epsilon,ST,cbar,LT,S,V_tot,da,de,dr,P,Q,R)

A = [-1.4 * beta;
     -0.59 - 3.1 * (ST * LT / (S * cbar)) * (alpha - epsilon);
     (1 - alpha * 180 / (15*pi)) * beta];

B = [-11    0                               5;
     0     -4.03 * (ST * LT^2) / (S * cbar^2)  0;
     1.7    0                               -11.5];

C = [-0.6   0                               0.22;
     0      -3.1 * (ST * LT) / (S * cbar)      0;
     0      0                               -0.63];

rot_rate = [P;
            Q;
            R];

control = [da;
           de;
           dr];

coef = A + B * (cbar/V_tot) * rot_rate + C * control; 

Cl = coef(1);
Cm = coef(2);
Cn = coef(3);

== matlab function Aircraft6DOFTrim/Aircraft Model/Aerodynamics/Moment Calculations ==
  data: Cl input; L_roll output; Cm input; Cn input; q_bar input; S input; cbar input; M_pitch output; N_yaw output; L input; D input; Y input; alpha input; cg input; ac input
function [L_roll,M_pitch,N_yaw] = fcn(Cl,Cm,Cn,q_bar,S,cbar,L,D,Y,alpha,cg,ac)

L_roll_ac = Cl * q_bar * S * cbar;   % rolling moment 

M_pitch_ac = Cm * q_bar * S * cbar;    % pitching moment 

N_yaw_ac = Cn * q_bar * S * cbar;   % yawing moment 

FA_s = [-D;
         Y;
        -L];

C_bs = [cos(alpha)  0   -sin(alpha);
        0           1   0;
        sin(alpha)  0   cos(alpha)];

FA_b = C_bs * FA_s;

MAac_b = [L_roll_ac;
          M_pitch_ac;
          N_yaw_ac];

MAcg_b = MAac_b + cross(FA_b,cg-ac);

L_roll = MAcg_b(1);

M_pitch = MAcg_b(2);

N_yaw = MAcg_b(3);

== matlab function Aircraft6DOFTrim/Aircraft Model/Aerodynamics/Aerodynamic Force in Body-axes ==
  data: L input; Fx output; D input; Y input; alpha input; beta input; Fy output; Fz output
function [Fx,Fy,Fz] = fcn(L,D,Y,alpha,beta)

Fx = L * sin(alpha) - D * cos(alpha) * cos(beta) - Y * cos(alpha) * sin(beta);

Fy = -D * sin(beta) + Y * cos(beta);

Fz = -L * cos(alpha) - D * sin(alpha) * cos(beta) - Y * sin(alpha) * sin(beta);

== matlab function Aircraft6DOFTrim/Aircraft Model/Engine Model /Engine Moments ==
  data: Fx_engine1 input; M output; Fx_engine2 input; engArm1 input; engArm2 input
function M = fcn(Fx_engine1,Fx_engine2,engArm1,engArm2)

F_engine1 = [Fx_engine1;
             0;
             0];

F_engine2 = [Fx_engine2;
             0;
             0];

M_engine1 = cross(engArm1,F_engine1);
M_engine2 = cross(engArm2,F_engine2);

M = M_engine1 + M_engine2;

== matlab function Aircraft6DOFTrim/Aircraft Model/6DOF EOM/vertical load factor ==
  data: Fz input; Nz output; mass input; g input
function Nz = fcn(Fz,mass,g)

Nz = -Fz/(mass * g);

== matlab function Aircraft6DOFTrim/Aircraft Model/Aerodynamics/Aerodynamic Force ==
  data: CL input; L output; CD input; CY input; q_bar input; S input; D output; Y output
function [L,D,Y] = fcn(CL,CD,CY,q_bar,S)

L = CL * q_bar * S;
D = CD * q_bar * S;
Y = CY * q_bar * S;

== matlab function Aircraft6DOFTrim/Aircraft Model/Aerodynamics/Aerodynamic Coefficients ==
  data: a0 input; a1 input; a2 input; a3 input; alpha input; CL output; alpha0 input; alpha_stall input; CLa input; beta input; ST input; S input; LT input; epsilon input; Q input; V_tot input; de input; CD output; CY output; dr input
function [CL,CD,CY] = fcn(a0,a1,a2,a3,alpha,alpha0,alpha_stall,CLa,beta,...
                          ST,S,LT,epsilon,Q,V_tot,de,dr)

% lift
if alpha <= alpha_stall
    CL_wb = CLa * (alpha - alpha0); % lift coefficient of the wing/body
else
    CL_wb = a0 + a1 * alpha + a2 * alpha^2 + a3 * alpha^3;
end
alpha_t = alpha - epsilon + de + 1.3 * (Q * LT)/ V_tot; % aoa of the tail

CL_t = ST/S * 3.1 * alpha_t;    % lift coefficient of the tail

CL = CL_wb + CL_t;

% drag
CD = 0.13 + 0.07 * (CL_wb - 0.45)^2;
%CD = 0.13 + 0.07 * (CLa * alpha + 0.654)^2;

% sideforce
CY = -1.6 * beta + 0.24 * dr;

== matlab function Aircraft6DOFTrim/Aircraft Model/6DOF EOM/Force Equations ==
  data: U input; V input; U_dot output; V_dot output; W input; P input; Q input; R input; Fx input; Fy input; Fz input; phi input; theta input; m input; g input; W_dot output
function [U_dot,V_dot,W_dot] = fcn(U,V,W,P,Q,R,Fx,Fy,Fz,phi,theta,m,g)

U_dot = R * V - Q * W - g * sin(theta) + Fx / m;

V_dot = -R * U + P * W + g * sin(phi) * cos(theta) + Fy / m;

W_dot = Q * U - P * V + g * cos(phi) * cos(theta) + Fz / m;

== matlab function Aircraft6DOFTrim/Aircraft Model/6DOF EOM/Kinematic Equations ==
  data: P input; phi_dot output; Q input; R input; phi input; theta input; theta_dot output; psi_dot output
function [phi_dot,theta_dot,psi_dot] = fcn(P,Q,R,phi,theta)

phi_dot = P + tan(theta) * (Q * sin(phi) + R * cos(phi));
theta_dot = Q * cos(phi) - R * sin(phi);
psi_dot = (Q * sin(phi) + R * cos(phi)) /  cos(theta);

== matlab function Aircraft6DOFTrim/Aircraft Model/6DOF EOM/Moment Equations ==
  data: c input; P_dot output; P input; Q input; R input; L_roll input; M_pitch input; N_yaw input; Q_dot output; R_dot output; Mxyz_engines input
function [P_dot,Q_dot,R_dot] = fcn(c,P,Q,R,L_roll,M_pitch,N_yaw,Mxyz_engines)

L_roll = L_roll + Mxyz_engines(1);
M_pitch = M_pitch + Mxyz_engines(2);
N_yaw = N_yaw + Mxyz_engines(3);

P_dot = (c(1) * R + c(2) * P) * Q + c(3) * L_roll + c(4) * N_yaw;

Q_dot = c(5) * P * R - c(6) * (P^2 - R^2) + c(7) * M_pitch;

R_dot = (c(8) * P - c(2) * R) * Q + c(4) * L_roll + c(9) * N_yaw;
